simulink model "x20240109_HVDCMMCInterconnection"  (R2023b)
settings: Solver=FixedStepDiscrete  StartTime=0.0  StopTime=2  FixedStep=Ts_Power  RelTol=1e-4  EnableMultiTasking=on
PreLoadFcn:
  | HVDCMMCInterconnectionParam
StartFcn:
  | tic
StopFcn:
  | toc
values from neighbouring files (symbols this model uses):
  C_PM = 1.758e-3    (= 0.001758)    [HVDCMMCInterconnectionParam.m]
  Cg = 50e-9    (= 5e-08)    [HVDCMMCInterconnectionParam.m]
  D_R = 0.001    [HVDCMMCInterconnectionParam.m]
  D_Rs = 1e8    (= 100000000)    [HVDCMMCInterconnectionParam.m]
  D_Vf = 0    [HVDCMMCInterconnectionParam.m]
  Fnom = 50    [HVDCMMCInterconnectionParam.m]
  HRM = 2    [HVDCMMCInterconnectionParam.m]
  Ki_Ireg = 6    [HVDCMMCInterconnectionParam.m]
  Ki_Preg = 1.0    (= 1)    [HVDCMMCInterconnectionParam.m]
  Ki_Qreg = 1.0    (= 1)    [HVDCMMCInterconnectionParam.m]
  Ki_VDCreg = 100    [HVDCMMCInterconnectionParam.m]
  Kp_Ireg = 0.6    [HVDCMMCInterconnectionParam.m]
  Kp_Preg = 0.5/3    (= 0.166666666667)    [HVDCMMCInterconnectionParam.m]
  Kp_Qreg = 0.5/3    (= 0.166666666667)    [HVDCMMCInterconnectionParam.m]
  Kp_VDCreg = 4    [HVDCMMCInterconnectionParam.m]
  L_cable = 15e-3    (= 0.015)    [HVDCMMCInterconnectionParam.m]
  Larm = Larm_pu*(Zb_ac/(2*pi*Fnom))    [HVDCMMCInterconnectionParam.m]
  Lff = Larm_pu/2    (= 0.075)    [HVDCMMCInterconnectionParam.m]
  Limits_Ireg = [ 2.0  -2.0]    [HVDCMMCInterconnectionParam.m]
  Limits_Preg = [ 1.2, 0.8 ]    [HVDCMMCInterconnectionParam.m]
  Limits_Qreg = [ 0.25, -0.25 ]    [HVDCMMCInterconnectionParam.m]
  Limits_VDCreg = [ 2.0  -2.0]    [HVDCMMCInterconnectionParam.m]
  Lxfo = 0.12    [HVDCMMCInterconnectionParam.m]
  Nb_PM = 36    [HVDCMMCInterconnectionParam.m]
  Pnom = 1000e6    (= 1000000000)    [HVDCMMCInterconnectionParam.m]
  R_cable = 0.5    [HVDCMMCInterconnectionParam.m]
  R_startup = 400    [HVDCMMCInterconnectionParam.m]
  Rarm = Rarm_pu*Zb_ac    [HVDCMMCInterconnectionParam.m]
  Rff = Rarm_pu/2    (= 0.00075)    [HVDCMMCInterconnectionParam.m]
  Rg = 100    [HVDCMMCInterconnectionParam.m]
  Rxfo = 0.003    [HVDCMMCInterconnectionParam.m]
  Slope_Pref = 0.5    [HVDCMMCInterconnectionParam.m]
  Slope_Qref = 0.5    [HVDCMMCInterconnectionParam.m]
  Slope_Vdc_ref = Vnom_dc/5    (= 128000)    [HVDCMMCInterconnectionParam.m]
  Tbrk1_On = 0.1    [HVDCMMCInterconnectionParam.m]
  Tbrk2_On = 1.0    (= 1)    [HVDCMMCInterconnectionParam.m]
  Tdeblock = 1.5    [HVDCMMCInterconnectionParam.m]
  Tfault = 9999    [HVDCMMCInterconnectionParam.m]
  Ton_Converter2 = 4    [HVDCMMCInterconnectionParam.m]
  Ton_PQreg = 4    [HVDCMMCInterconnectionParam.m]
  Ton_VDCreg = 1.5    [HVDCMMCInterconnectionParam.m]
  Ts = Ts_Control    (= 4e-05)    [HVDCMMCInterconnectionParam.m]
  Ts_Control = 40e-6    (= 4e-05)    [HVDCMMCInterconnectionParam.m]
  Ts_Power = 20e-6    (= 2e-05)    [HVDCMMCInterconnectionParam.m]
  Vb_ac = sqrt(2/3)*Vnom_sec    [HVDCMMCInterconnectionParam.m]
  Vb_dc = Vnom_dc    (= 640000)    [HVDCMMCInterconnectionParam.m]
  Vc0_PM = 0    [HVDCMMCInterconnectionParam.m]
  Vnom_dc = 640e3    (= 640000)    [HVDCMMCInterconnectionParam.m]
  Vnom_prim = 400e3    (= 400000)    [HVDCMMCInterconnectionParam.m]
  Vnom_sec = 333e3    (= 333000)    [HVDCMMCInterconnectionParam.m]
  w = 2*pi*Fnom    (= 314.159265359)    [HVDCMMCInterconnectionParam.m]
undefined symbols (not defined in the file or in its folder): DiscIntNeverNeededParam, gcbh, Pcc, S, sps_AC, sps_ACDC2, sps_rtmsupport
libraries: simulink x48, spsControlledVoltageSourceLib x30, spsCurrentMeasurementLib x30, MMC_Lib x30, spsDiodeLib x20, spsSeriesRLCBranchLib x14, powerlib_extras x12, spsVoltageMeasurementLib x12, spsSecondOrderFilterLib x8, spsabctodq0Lib x8, spsGroundLib x7, spsMeanLib x4
(part 3 of 9)

== system x20240109_HVDCMMCInterconnection/Gates ==
  Gain : Gain  Gain=0
  Mux : Mux  Inputs=[1 1 1 1 1 1 1 1 1 1 1 1 1 1]
  gates : Outport  VectorParamsAs1DForOutWhenUnconnected=off
  wires:
  Mux/1 -> Gain/1
  [T47_4275_3649146433913] -> Mux/1
  [T48_4324_3649669992407] -> Mux/2
  [T40_3529_2249035564301] -> Mux/3
  [T40_3547_2353536747378] -> Mux/4
  [T40_3533_2265623233840] -> Mux/5
  [T41_3600_2390188926951] -> Mux/6
  [T40_3531_2249723496385] -> Mux/7
  [T40_3549_2354145301308] -> Mux/8
  [T40_3535_2266295809333] -> Mux/9
  [T40_3553_2370553433949] -> Mux/10
  [T40_3533_2250552886404] -> Mux/11
  [T40_3551_2354895313173] -> Mux/12
  [T40_3537_2267109842763] -> Mux/13
  [T40_3555_2371288089224] -> Mux/14
  Gain/1 -> gates/1
